simulink model "Problem3"  (R2020b)
settings: Solver=VariableStepAuto  StartTime=0.0  StopTime=10.0  RelTol=1e-3
PreLoadFcn:
  | clear all;
  | close all;
  | clc;
  | m=1000;
  | b=50;
  | u=500;
settings Model: Creator=omkar  LastModifiedBy=omkar

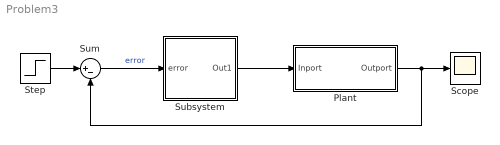
== system Problem3 ==
  Plant : Subsystem
  Scope : Scope
  Step : Step  Time=0  After=u  SampleTime=0
  Subsystem : Subsystem
      settings: MinAlgLoopOccurrences=on
  Sum : Sum  Inputs=|+-
  wires:
  Subsystem/1(Out1) -> Plant/1(Inport)
  Plant/1(Outport) -> Scope/1, Sum/2
  Step/1 -> Sum/1
  Sum/1 -> Subsystem/1(error)  "error"

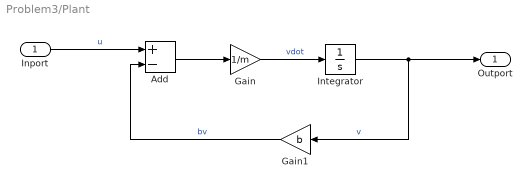
== system Problem3/Plant ==
  Inport : Inport
  Add : Sum  Inputs=+-
  Gain : Gain  Gain=1/m
  Gain1 : Gain  Gain=b
  Integrator : Integrator
  Outport : Outport
  wires:
  Inport/1 -> Add/1  "u"
  Gain/1 -> Integrator/1  "vdot"
  Integrator/1 -> Gain1/1, Outport/1  "v"
  Add/1 -> Gain/1
  Gain1/1 -> Add/2  "bv"

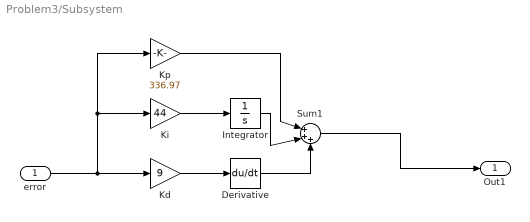
== system Problem3/Subsystem ==
  error : Inport  OutDataTypeStr=double  PortDimensions=1  SampleTime=0
  Derivative : Derivative
  Integrator : Integrator
  Kd : Gain  Gain=9
  Ki : Gain  Gain=44
  Kp : Gain  Gain=336.97
  Sum1 : Sum  Inputs=|+++
  Out1 : Outport  OutDataTypeStr=double  PortDimensions=1  SampleTime=0
  wires:
  Sum1/1 -> Out1/1
  Kp/1 -> Sum1/1
  Kd/1 -> Derivative/1
  error/1 -> Kp/1, Ki/1, Kd/1
  Derivative/1 -> Sum1/3
  Integrator/1 -> Sum1/2
  Ki/1 -> Integrator/1
